simulink subsystem "modulador_tension"  (R2023b)
settings: Solver=VariableStepAuto  StartTime=0.0  StopTime=10.0  RelTol=1e-3
settings Model: Creator=rodri  LastModifiedBy=nahue

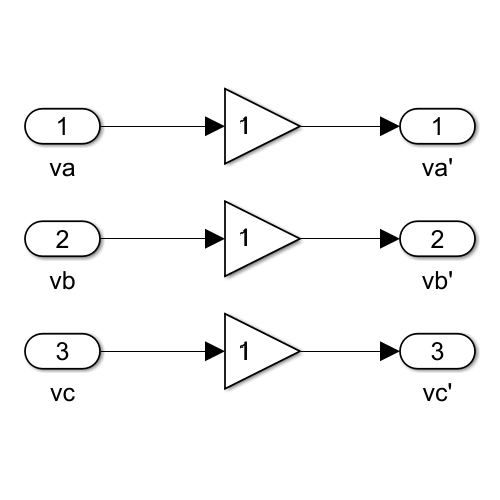
[thumbnail: Simulink's stored preview of the top-level diagram]
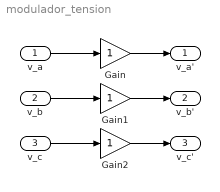
== system modulador_tension ==
  v_a : Inport
  v_b : Inport  Port=2
  v_c : Inport  Port=3
  Gain : Gain
  Gain1 : Gain
  Gain2 : Gain
  v_a' : Outport
  v_b' : Outport  Port=2
  v_c' : Outport  Port=3
  wires:
  v_a/1 -> Gain/1
  Gain/1 -> v_a'/1
  Gain1/1 -> v_b'/1
  v_b/1 -> Gain1/1
  Gain2/1 -> v_c'/1
  v_c/1 -> Gain2/1
